simulink model "Question_6_b"  (R2014a)
settings: Solver=ode45  StartTime=0.0  StopTime=10.0  RelTol=1e-3
settings Model: Creator=Shiyu  LastModifiedBy=Shiyu

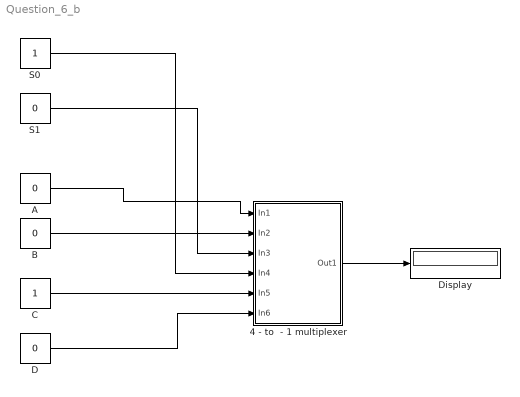
== system Question_6_b ==
  4 - to  - 1 multiplexer : Subsystem
  A : Constant  Value=0
  B : Constant  Value=0
  C : Constant
  D : Constant  Value=0
  Display : Display
  S0 : Constant
  S1 : Constant  Value=0
  wires:
  A/1 -> 4 - to  - 1 multiplexer/1(In1)
  B/1 -> 4 - to  - 1 multiplexer/2(In2)
  S1/1 -> 4 - to  - 1 multiplexer/3(In3)
  S0/1 -> 4 - to  - 1 multiplexer/4(In4)
  C/1 -> 4 - to  - 1 multiplexer/5(In5)
  D/1 -> 4 - to  - 1 multiplexer/6(In6)
  4 - to  - 1 multiplexer/1(Out1) -> Display/1

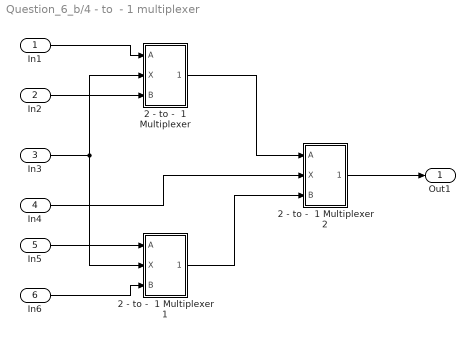
== system Question_6_b/4 - to  - 1 multiplexer ==
  In1 : Inport
  In2 : Inport  Port=2
  In3 : Inport  Port=3
  In4 : Inport  Port=4
  In5 : Inport  Port=5
  In6 : Inport  Port=6
  "2 - to -  1 Multiplexer " : Subsystem
  2 - to -  1 Multiplexer 1 : Subsystem
  2 - to -  1 Multiplexer 2 : Subsystem
  Out1 : Outport
  wires:
  In4/1 -> 2 - to -  1 Multiplexer 2/2(X)
  In1/1 -> "2 - to -  1 Multiplexer "/1(A)
  In3/1 -> 2 - to -  1 Multiplexer 1/2(X), "2 - to -  1 Multiplexer "/2(X)
  In5/1 -> 2 - to -  1 Multiplexer 1/1(A)
  2 - to -  1 Multiplexer 2/1(Out1) -> Out1/1
  In2/1 -> "2 - to -  1 Multiplexer "/3(B)
  In6/1 -> 2 - to -  1 Multiplexer 1/3(B)
  "2 - to -  1 Multiplexer "/1(Out1) -> 2 - to -  1 Multiplexer 2/1(A)
  2 - to -  1 Multiplexer 1/1(Out1) -> 2 - to -  1 Multiplexer 2/3(B)

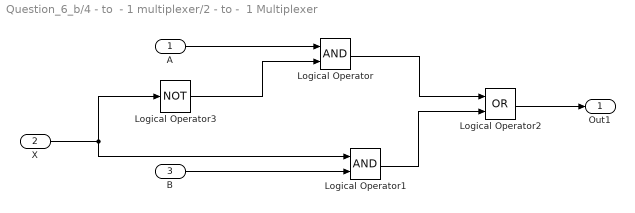
== system Question_6_b/4 - to  - 1 multiplexer/2 - to -  1 Multiplexer  ==
  A : Inport
  X : Inport  Port=2
  B : Inport  Port=3
  Logical Operator : Logic  AllPortsSameDT=off  OutDataTypeStr=boolean
  Logical Operator1 : Logic  AllPortsSameDT=off  OutDataTypeStr=boolean
  Logical Operator2 : Logic  Operator=OR  AllPortsSameDT=off  OutDataTypeStr=boolean
  Logical Operator3 : Logic  Operator=NOT  AllPortsSameDT=off  OutDataTypeStr=boolean
  Out1 : Outport
  wires:
  Logical Operator3/1 -> Logical Operator/2
  A/1 -> Logical Operator/1
  X/1 -> Logical Operator3/1, Logical Operator1/1
  B/1 -> Logical Operator1/2
  Logical Operator/1 -> Logical Operator2/1
  Logical Operator2/1 -> Out1/1
  Logical Operator1/1 -> Logical Operator2/2

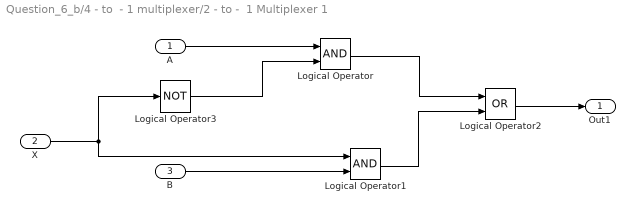
== system Question_6_b/4 - to  - 1 multiplexer/2 - to -  1 Multiplexer 1 ==
  A : Inport
  X : Inport  Port=2
  B : Inport  Port=3
  Logical Operator : Logic  AllPortsSameDT=off  OutDataTypeStr=boolean
  Logical Operator1 : Logic  AllPortsSameDT=off  OutDataTypeStr=boolean
  Logical Operator2 : Logic  Operator=OR  AllPortsSameDT=off  OutDataTypeStr=boolean
  Logical Operator3 : Logic  Operator=NOT  AllPortsSameDT=off  OutDataTypeStr=boolean
  Out1 : Outport
  wires:
  Logical Operator3/1 -> Logical Operator/2
  A/1 -> Logical Operator/1
  X/1 -> Logical Operator3/1, Logical Operator1/1
  B/1 -> Logical Operator1/2
  Logical Operator/1 -> Logical Operator2/1
  Logical Operator2/1 -> Out1/1
  Logical Operator1/1 -> Logical Operator2/2

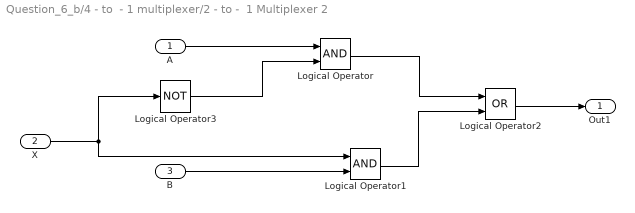
== system Question_6_b/4 - to  - 1 multiplexer/2 - to -  1 Multiplexer 2 ==
  A : Inport
  X : Inport  Port=2
  B : Inport  Port=3
  Logical Operator : Logic  AllPortsSameDT=off  OutDataTypeStr=boolean
  Logical Operator1 : Logic  AllPortsSameDT=off  OutDataTypeStr=boolean
  Logical Operator2 : Logic  Operator=OR  AllPortsSameDT=off  OutDataTypeStr=boolean
  Logical Operator3 : Logic  Operator=NOT  AllPortsSameDT=off  OutDataTypeStr=boolean
  Out1 : Outport
  wires:
  Logical Operator3/1 -> Logical Operator/2
  A/1 -> Logical Operator/1
  X/1 -> Logical Operator3/1, Logical Operator1/1
  B/1 -> Logical Operator1/2
  Logical Operator/1 -> Logical Operator2/1
  Logical Operator2/1 -> Out1/1
  Logical Operator1/1 -> Logical Operator2/2
